simulink model "Dynamic"  (R2016b)
settings: Solver=ode5  StartTime=0.0  StopTime=inf  FixedStep=1e-4  RelTol=1e-3
settings Model: Creator=Admin  LastModifiedBy=Admin

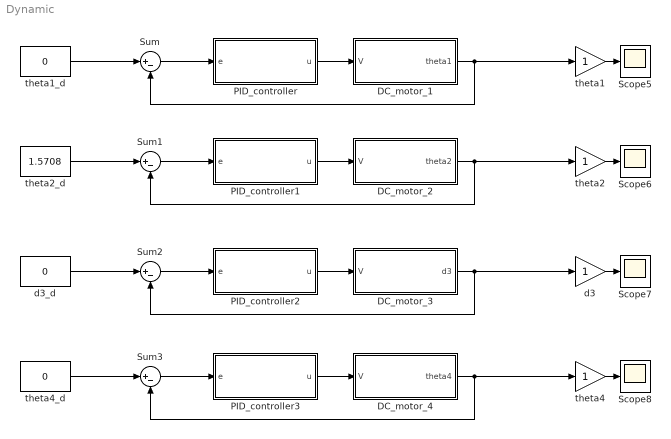
== system Dynamic ==
  DC_motor_1 : Subsystem  mask{Ki=0.043, Kb=0.04297, L=0.0001, R=1.025, Jeff=0.000056+(1e-4)*5, Beff=0.00008092, N=100}
  DC_motor_2 : Subsystem  mask{Ki=0.043, Kb=0.04297, L=0.0001, R=1.025, Jeff=0.000056+(1e-4)*5, Beff=0.00008092, N=100}
  DC_motor_3 : Subsystem  mask{Ki=0.043, Kb=0.04297, L=0.0001, R=1.025, Jeff=0.000056+(1e-4)*5, Beff=0.00008092, N=50}
  DC_motor_4 : Subsystem  mask{Ki=0.043, Kb=0.04297, L=0.0001, R=1.025, Jeff=0.000056+(1e-4)*5, Beff=0.00008092, N=100}
  PID_controller : Subsystem  mask{Kp=350, Ki=0, Kd=50}
  PID_controller1 : Subsystem  mask{Kp=350, Ki=0, Kd=50}
  PID_controller2 : Subsystem  mask{Kp=350, Ki=0, Kd=50}
  PID_controller3 : Subsystem  mask{Kp=350, Ki=0, Kd=50}
  Scope{5..8} (4 alike) : Scope
  Sum{,1..3} (4 alike) : Sum  Inputs=|+-
  d3 : Gain
  d3_d : Constant  Value=0
  theta1 : Gain
  theta1_d : Constant  Value=0
  theta2 : Gain
  theta2_d : Constant  Value=1.5708
  theta4 : Gain
  theta4_d : Constant  Value=0
  wires:
  DC_motor_1/1(theta1) -> Sum/2, theta1/1
  Sum/1 -> PID_controller/1(e)
  PID_controller/1(u) -> DC_motor_1/1(V)
  DC_motor_2/1(theta2) -> Sum1/2, theta2/1
  Sum1/1 -> PID_controller1/1(e)
  PID_controller1/1(u) -> DC_motor_2/1(V)
  Sum2/1 -> PID_controller2/1(e)
  PID_controller2/1(u) -> DC_motor_3/1(V)
  DC_motor_4/1(theta4) -> Sum3/2, theta4/1
  Sum3/1 -> PID_controller3/1(e)
  PID_controller3/1(u) -> DC_motor_4/1(V)
  theta1_d/1 -> Sum/1
  DC_motor_3/1(d3) -> Sum2/2, d3/1
  theta2_d/1 -> Sum1/1
  d3_d/1 -> Sum2/1
  theta4_d/1 -> Sum3/1
  theta1/1 -> Scope5/1
  theta2/1 -> Scope6/1
  d3/1 -> Scope7/1
  theta4/1 -> Scope8/1

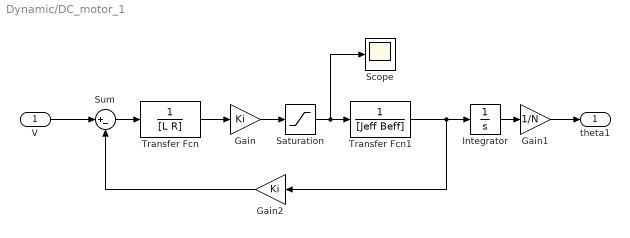
== system Dynamic/DC_motor_1 ==
  V : Inport
  Gain : Gain  Gain=Ki
  Gain1 : Gain  Gain=1/N
  Gain2 : Gain  Gain=Ki
  Integrator : Integrator
  Saturation : Saturate  UpperLimit=4  LowerLimit=-4
  Scope : Scope
  Sum : Sum  Inputs=|+-
  Transfer Fcn : TransferFcn  Denominator=[L R]
  Transfer Fcn1 : TransferFcn  Denominator=[Jeff Beff]
  theta1 : Outport
  wires:
  Sum/1 -> Transfer Fcn/1
  Transfer Fcn/1 -> Gain/1
  Gain/1 -> Saturation/1
  Transfer Fcn1/1 -> Integrator/1, Gain2/1
  Integrator/1 -> Gain1/1
  Gain1/1 -> theta1/1
  Gain2/1 -> Sum/2
  V/1 -> Sum/1
  Saturation/1 -> Scope/1, Transfer Fcn1/1

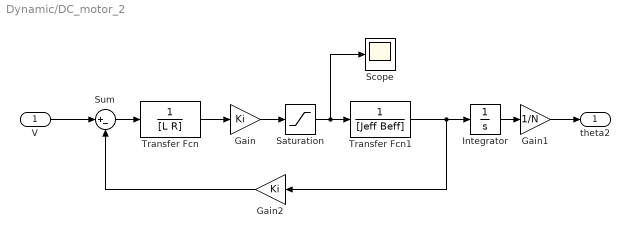
== system Dynamic/DC_motor_2 ==
  V : Inport
  Gain : Gain  Gain=Ki
  Gain1 : Gain  Gain=1/N
  Gain2 : Gain  Gain=Ki
  Integrator : Integrator
  Saturation : Saturate  UpperLimit=4  LowerLimit=-4
  Scope : Scope
  Sum : Sum  Inputs=|+-
  Transfer Fcn : TransferFcn  Denominator=[L R]
  Transfer Fcn1 : TransferFcn  Denominator=[Jeff Beff]
  theta2 : Outport
  wires:
  Sum/1 -> Transfer Fcn/1
  Transfer Fcn/1 -> Gain/1
  Gain/1 -> Saturation/1
  Transfer Fcn1/1 -> Integrator/1, Gain2/1
  Integrator/1 -> Gain1/1
  Gain1/1 -> theta2/1
  Gain2/1 -> Sum/2
  V/1 -> Sum/1
  Saturation/1 -> Scope/1, Transfer Fcn1/1

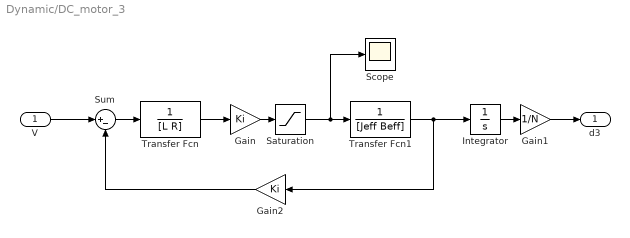
== system Dynamic/DC_motor_3 ==
  V : Inport
  Gain : Gain  Gain=Ki
  Gain1 : Gain  Gain=1/N
  Gain2 : Gain  Gain=Ki
  Integrator : Integrator
  Saturation : Saturate  UpperLimit=4  LowerLimit=-4
  Scope : Scope
  Sum : Sum  Inputs=|+-
  Transfer Fcn : TransferFcn  Denominator=[L R]
  Transfer Fcn1 : TransferFcn  Denominator=[Jeff Beff]
  d3 : Outport
  wires:
  Sum/1 -> Transfer Fcn/1
  Transfer Fcn/1 -> Gain/1
  Gain/1 -> Saturation/1
  Transfer Fcn1/1 -> Integrator/1, Gain2/1
  Integrator/1 -> Gain1/1
  Gain1/1 -> d3/1
  Gain2/1 -> Sum/2
  V/1 -> Sum/1
  Saturation/1 -> Scope/1, Transfer Fcn1/1

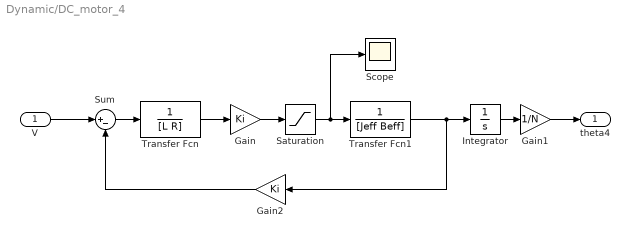
== system Dynamic/DC_motor_4 ==
  V : Inport
  Gain : Gain  Gain=Ki
  Gain1 : Gain  Gain=1/N
  Gain2 : Gain  Gain=Ki
  Integrator : Integrator
  Saturation : Saturate  UpperLimit=4  LowerLimit=-4
  Scope : Scope
  Sum : Sum  Inputs=|+-
  Transfer Fcn : TransferFcn  Denominator=[L R]
  Transfer Fcn1 : TransferFcn  Denominator=[Jeff Beff]
  theta4 : Outport
  wires:
  Sum/1 -> Transfer Fcn/1
  Transfer Fcn/1 -> Gain/1
  Gain/1 -> Saturation/1
  Transfer Fcn1/1 -> Integrator/1, Gain2/1
  Integrator/1 -> Gain1/1
  Gain1/1 -> theta4/1
  Gain2/1 -> Sum/2
  V/1 -> Sum/1
  Saturation/1 -> Scope/1, Transfer Fcn1/1

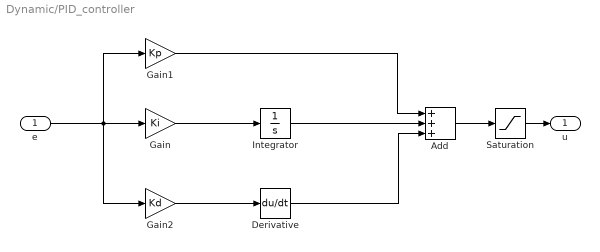
== system Dynamic/PID_controller ==
  e : Inport
  Add : Sum  Inputs=+++
  Derivative : Derivative
  Gain : Gain  Gain=Ki
  Gain1 : Gain  Gain=Kp
  Gain2 : Gain  Gain=Kd
  Integrator : Integrator
  Saturation : Saturate  UpperLimit=48  LowerLimit=-48
  u : Outport
  wires:
  e/1 -> Gain2/1, Gain1/1, Gain/1
  Gain/1 -> Integrator/1
  Gain2/1 -> Derivative/1
  Gain1/1 -> Add/1
  Integrator/1 -> Add/2
  Derivative/1 -> Add/3
  Add/1 -> Saturation/1
  Saturation/1 -> u/1

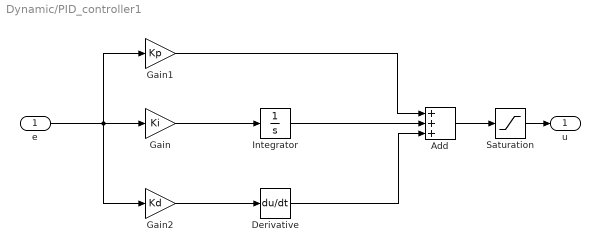
== system Dynamic/PID_controller1 ==
  e : Inport
  Add : Sum  Inputs=+++
  Derivative : Derivative
  Gain : Gain  Gain=Ki
  Gain1 : Gain  Gain=Kp
  Gain2 : Gain  Gain=Kd
  Integrator : Integrator
  Saturation : Saturate  UpperLimit=48  LowerLimit=-48
  u : Outport
  wires:
  e/1 -> Gain2/1, Gain1/1, Gain/1
  Gain/1 -> Integrator/1
  Gain2/1 -> Derivative/1
  Gain1/1 -> Add/1
  Integrator/1 -> Add/2
  Derivative/1 -> Add/3
  Add/1 -> Saturation/1
  Saturation/1 -> u/1

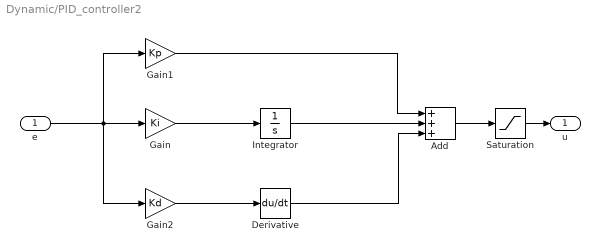
== system Dynamic/PID_controller2 ==
  e : Inport
  Add : Sum  Inputs=+++
  Derivative : Derivative
  Gain : Gain  Gain=Ki
  Gain1 : Gain  Gain=Kp
  Gain2 : Gain  Gain=Kd
  Integrator : Integrator
  Saturation : Saturate  UpperLimit=48  LowerLimit=-48
  u : Outport
  wires:
  e/1 -> Gain2/1, Gain1/1, Gain/1
  Gain/1 -> Integrator/1
  Gain2/1 -> Derivative/1
  Gain1/1 -> Add/1
  Integrator/1 -> Add/2
  Derivative/1 -> Add/3
  Add/1 -> Saturation/1
  Saturation/1 -> u/1

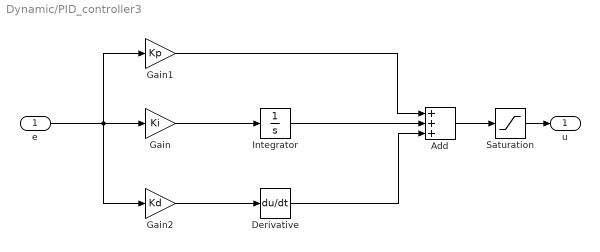
== system Dynamic/PID_controller3 ==
  e : Inport
  Add : Sum  Inputs=+++
  Derivative : Derivative
  Gain : Gain  Gain=Ki
  Gain1 : Gain  Gain=Kp
  Gain2 : Gain  Gain=Kd
  Integrator : Integrator
  Saturation : Saturate  UpperLimit=48  LowerLimit=-48
  u : Outport
  wires:
  e/1 -> Gain2/1, Gain1/1, Gain/1
  Gain/1 -> Integrator/1
  Gain2/1 -> Derivative/1
  Gain1/1 -> Add/1
  Integrator/1 -> Add/2
  Derivative/1 -> Add/3
  Add/1 -> Saturation/1
  Saturation/1 -> u/1
